simulink model "Sinusoidal_Road"  (R2023b)
settings: Solver=VariableStepAuto  StartTime=0.0  StopTime=10  RelTol=1e-3
values from neighbouring files (symbols this model uses):
  A = [0.01, 0.05, 0.1]    [Parameters.m]
  a = 1.35    [Parameters.m]
  b = 1.5    [Parameters.m]
  g = 9.81    [Parameters.m]
  I = 650    [Parameters.m]
  Kt = 14e4    (= 140000)    [Parameters.m]
  lambda = 1    [Parameters.m]
  Mw = 20    [Parameters.m]
  v = [1, 2, 3, 5, 8, 10]    [Parameters.m]
libraries: CarModelLibrary x6, simulink x4
settings Model: Creator=fb552  LastModifiedBy=franc
settings SolverCC: AlgebraicLoopSolver=TrustRegion
settings DebuggingCC: UnconnectedInputMsg=warning  UnconnectedOutputMsg=warning  UnconnectedLineMsg=warning
settings ModelReferenceCC: EnableRefExpFcnMdlSchedulingChecks=on

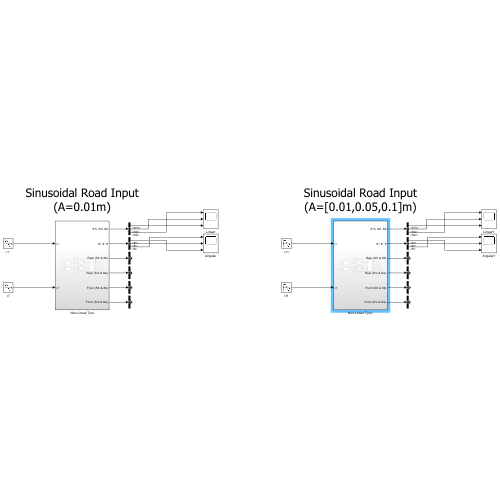
[thumbnail: Simulink's stored preview of the top-level diagram]
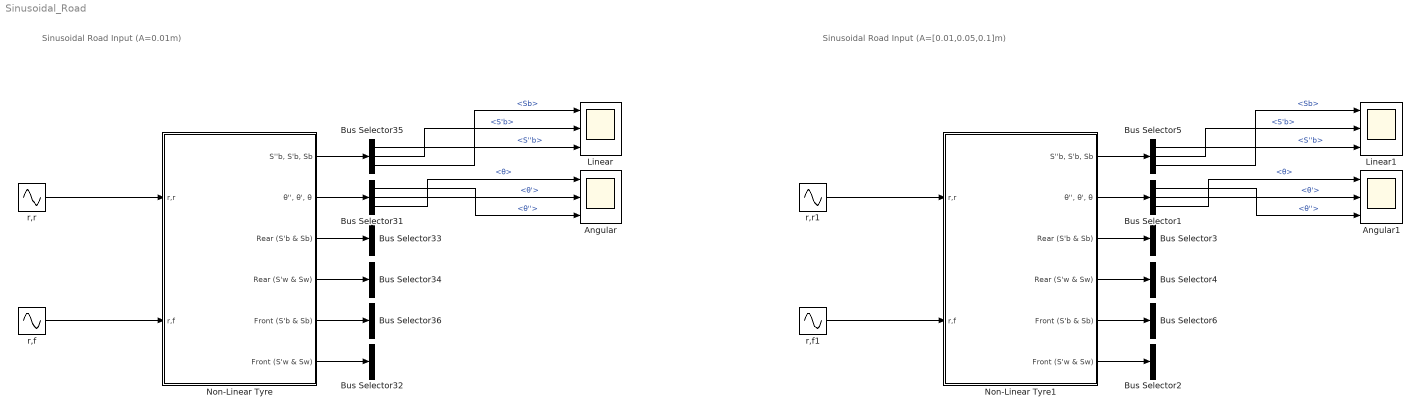
== system Sinusoidal_Road ==
  note: Sinusoidal Road Input (A=0.01m)
  note: Sinusoidal Road Input (A=[0.01,0.05,0.1]m)
  Angular : Scope  NumInputPorts=3
  Angular1 : Scope  NumInputPorts=3
  Bus Selector1 : BusSelector  OutputSignals=θ'',θ',θ
  Bus Selector{2,4,32,34} (4 alike) : BusSelector  OutputSignals=Sw
  Bus Selector{3,6,33,36} (4 alike) : BusSelector  OutputSignals=Sb
  Bus Selector31 : BusSelector  OutputSignals=θ'',θ',θ
  Bus Selector35 : BusSelector  OutputSignals=S''b,S'b,Sb
  Bus Selector5 : BusSelector  OutputSignals=S''b,S'b,Sb
  Linear : Scope  NumInputPorts=3
  Linear1 : Scope  NumInputPorts=3
  Non-Linear Tyre : Subsystem
  Non-Linear Tyre1 : Subsystem
  r,f : Sin  Amplitude=A(1)  Frequency=2*pi*(v/lambda)  SampleTime=0
  r,f1 : Sin  Amplitude=A  Frequency=2*pi*(v(end)/lambda)  SampleTime=0
  r,r : Sin  Amplitude=A(1)  Frequency=2*pi*(v/lambda)  Phase=(a+b)*2*pi  SampleTime=0
  r,r1 : Sin  Amplitude=A  Frequency=2*pi*(v(end)/lambda)  Phase=(a+b)*2*pi  SampleTime=0
  wires:
  Non-Linear Tyre/2("θ'', θ', θ") -> Bus Selector31/1
  Non-Linear Tyre/6(Front (S'w & Sw)) -> Bus Selector32/1
  Bus Selector35/3 -> Linear/1  "<Sb>"
  Non-Linear Tyre/4(Rear (S'w & Sw)) -> Bus Selector34/1
  Non-Linear Tyre/5(Front (S'b & Sb)) -> Bus Selector36/1
  Non-Linear Tyre/1("S''b, S'b, Sb") -> Bus Selector35/1
  Non-Linear Tyre/3(Rear (S'b & Sb)) -> Bus Selector33/1
  r,f/1 -> Non-Linear Tyre/2(r,f)
  r,r/1 -> Non-Linear Tyre/1(r,r)
  Bus Selector35/2 -> Linear/2  "<S'b>"
  Bus Selector35/1 -> Linear/3  "<S''b>"
  Bus Selector31/3 -> Angular/1  "<θ>"
  Bus Selector31/2 -> Angular/2  "<θ'>"
  Bus Selector31/1 -> Angular/3  "<θ''>"
  Non-Linear Tyre1/3(Rear (S'b & Sb)) -> Bus Selector3/1
  Bus Selector5/3 -> Linear1/1  "<Sb>"
  r,r1/1 -> Non-Linear Tyre1/1(r,r)
  Bus Selector5/2 -> Linear1/2  "<S'b>"
  r,f1/1 -> Non-Linear Tyre1/2(r,f)
  Non-Linear Tyre1/2("θ'', θ', θ") -> Bus Selector1/1
  Non-Linear Tyre1/4(Rear (S'w & Sw)) -> Bus Selector4/1
  Non-Linear Tyre1/5(Front (S'b & Sb)) -> Bus Selector6/1
  Bus Selector1/3 -> Angular1/1  "<θ>"
  Non-Linear Tyre1/1("S''b, S'b, Sb") -> Bus Selector5/1
  Bus Selector1/1 -> Angular1/3  "<θ''>"
  Bus Selector1/2 -> Angular1/2  "<θ'>"
  Non-Linear Tyre1/6(Front (S'w & Sw)) -> Bus Selector2/1
  Bus Selector5/1 -> Linear1/3  "<S''b>"

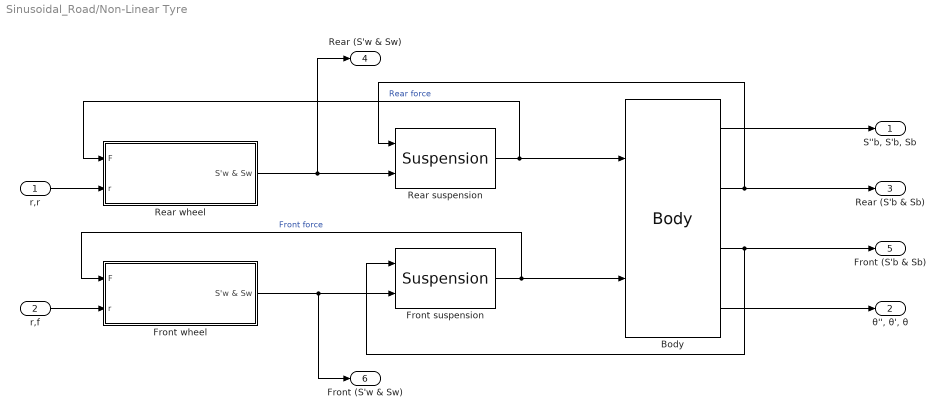
== system Sinusoidal_Road/Non-Linear Tyre ==
  r,r : Inport
  r,f : Inport  Port=2
  Body : CarModelLibrary/Body  mb=Mb  I=I  a=a  b=b
  Front suspension : CarModelLibrary/Suspension  ks=Ks  ksstiff=Kstiff  x0=x0  csb=Csc  csr=Cse
  Front wheel : Subsystem  AncestorBlock=CarModelLibrary/Wheel  mask{mw=Mw, Kt=Kt, g=g}
      mask prompts: mw "Wheel Mass (Kg)"; Kt "Tyre Stiffness"; g "Gravitational acceleration"
  Rear suspension : CarModelLibrary/Suspension  ks=Ks  ksstiff=Kstiff  x0=x0  csb=Csc  csr=Cse
  Rear wheel : Subsystem  AncestorBlock=CarModelLibrary/Wheel  mask{mw=Mw, Kt=Kt, g=g}
      mask prompts: mw "Wheel Mass (Kg)"; Kt "Tyre Stiffness"; g "Gravitational acceleration"
  "S''b, S'b, Sb" : Outport
  "θ'', θ', θ" : Outport  Port=2
  Rear (S'b & Sb) : Outport  Port=3
  Rear (S'w & Sw) : Outport  Port=4
  Front (S'b & Sb) : Outport  Port=5
  Front (S'w & Sw) : Outport  Port=6
  wires:
  Body/1 -> "S''b, S'b, Sb"/1
  Body/2 -> Rear suspension/1, Rear (S'b & Sb)/1
  Front wheel/1(S'w & Sw) -> Front suspension/2, Front (S'w & Sw)/1
  Rear wheel/1(S'w & Sw) -> Rear suspension/2, Rear (S'w & Sw)/1
  Body/4 -> "θ'', θ', θ"/1
  Body/3 -> Front suspension/1, Front (S'b & Sb)/1
  Rear suspension/1 -> Body/1, Rear wheel/1(F)  "Rear force"
  r,r/1 -> Rear wheel/2(r)
  r,f/1 -> Front wheel/2(r)
  Front suspension/1 -> Front wheel/1(F), Body/2  "Front force"

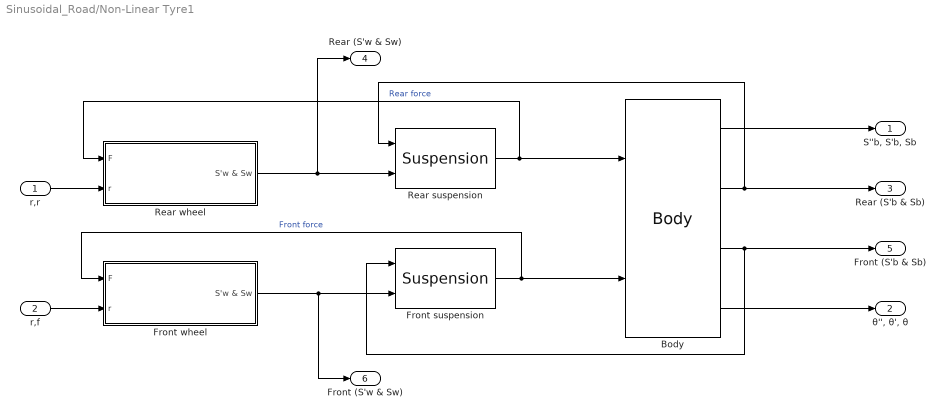
== system Sinusoidal_Road/Non-Linear Tyre1 ==
  r,r : Inport
  r,f : Inport  Port=2
  Body : CarModelLibrary/Body  mb=Mb  I=I  a=a  b=b
  Front suspension : CarModelLibrary/Suspension  ks=Ks  ksstiff=Kstiff  x0=x0  csb=Csc  csr=Cse
  Front wheel : Subsystem  AncestorBlock=CarModelLibrary/Wheel  mask{mw=Mw, Kt=Kt, g=g}
      mask prompts: mw "Wheel Mass (Kg)"; Kt "Tyre Stiffness"; g "Gravitational acceleration"
  Rear suspension : CarModelLibrary/Suspension  ks=Ks  ksstiff=Kstiff  x0=x0  csb=Csc  csr=Cse
  Rear wheel : Subsystem  AncestorBlock=CarModelLibrary/Wheel  mask{mw=Mw, Kt=Kt, g=g}
      mask prompts: mw "Wheel Mass (Kg)"; Kt "Tyre Stiffness"; g "Gravitational acceleration"
  "S''b, S'b, Sb" : Outport
  "θ'', θ', θ" : Outport  Port=2
  Rear (S'b & Sb) : Outport  Port=3
  Rear (S'w & Sw) : Outport  Port=4
  Front (S'b & Sb) : Outport  Port=5
  Front (S'w & Sw) : Outport  Port=6
  wires:
  Body/1 -> "S''b, S'b, Sb"/1
  Body/2 -> Rear suspension/1, Rear (S'b & Sb)/1
  Front wheel/1(S'w & Sw) -> Front suspension/2, Front (S'w & Sw)/1
  Rear wheel/1(S'w & Sw) -> Rear suspension/2, Rear (S'w & Sw)/1
  Body/4 -> "θ'', θ', θ"/1
  Body/3 -> Front suspension/1, Front (S'b & Sb)/1
  Rear suspension/1 -> Body/1, Rear wheel/1(F)  "Rear force"
  r,r/1 -> Rear wheel/2(r)
  r,f/1 -> Front wheel/2(r)
  Front suspension/1 -> Front wheel/1(F), Body/2  "Front force"

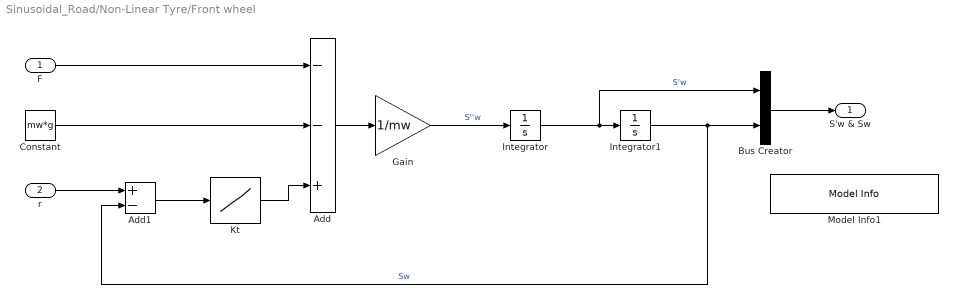
== system Sinusoidal_Road/Non-Linear Tyre/Front wheel ==
  F : Inport
  r : Inport  Port=2
  Add : Sum  Inputs=--+
  Add1 : Sum  Inputs=+-
  Bus Creator : BusCreator  Inputs=2
  Constant : Constant  Value=mw*g
  Gain : Gain  Gain=1/mw
  Integrator : Integrator
  Integrator1 : Integrator
  Kt : Lookup_n-D  NumberOfTableDimensions=1  BreakpointsForDimension1=[-1, 0, 1]  Table=[0, 0, Kt]  InternalRulePriority=Speed  RndMeth=Simplest
  Model Info1 : simulink/Model-Wide Utilities/Model Info  Frame=on  DisplayStringWithTags=m * S''w = -F + Kt (r-S) - m*g  HorizontalTextAlignment=Center  LeftAlignmentValue=0.5
  S'w & Sw : Outport
  wires:
  Kt/1 -> Add/3
  F/1 -> Add/1
  Constant/1 -> Add/2
  Gain/1 -> Integrator/1  "S''w"
  Add/1 -> Gain/1
  Integrator1/1 -> Add1/2, Bus Creator/2  "Sw"
  Bus Creator/1 -> S'w & Sw/1
  Integrator/1 -> Integrator1/1, Bus Creator/1  "S'w"
  Add1/1 -> Kt/1
  r/1 -> Add1/1

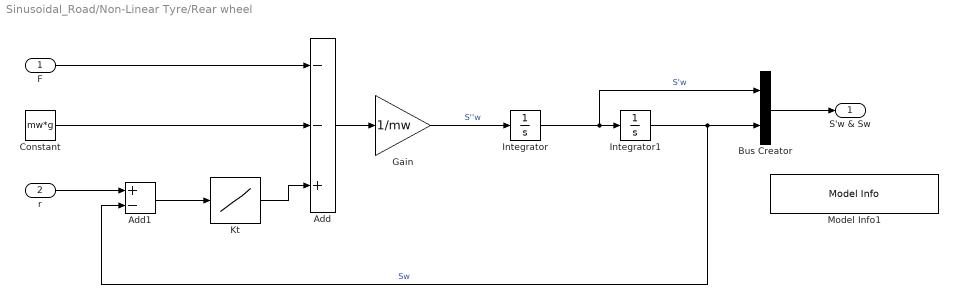
== system Sinusoidal_Road/Non-Linear Tyre/Rear wheel ==
  F : Inport
  r : Inport  Port=2
  Add : Sum  Inputs=--+
  Add1 : Sum  Inputs=+-
  Bus Creator : BusCreator  Inputs=2
  Constant : Constant  Value=mw*g
  Gain : Gain  Gain=1/mw
  Integrator : Integrator
  Integrator1 : Integrator
  Kt : Lookup_n-D  NumberOfTableDimensions=1  BreakpointsForDimension1=[-1, 0, 1]  Table=[0, 0, Kt]  InternalRulePriority=Speed  RndMeth=Simplest
  Model Info1 : simulink/Model-Wide Utilities/Model Info  Frame=on  DisplayStringWithTags=m * S''w = -F + Kt (r-S) - m*g  HorizontalTextAlignment=Center  LeftAlignmentValue=0.5
  S'w & Sw : Outport
  wires:
  Kt/1 -> Add/3
  F/1 -> Add/1
  Constant/1 -> Add/2
  Gain/1 -> Integrator/1  "S''w"
  Add/1 -> Gain/1
  Integrator1/1 -> Add1/2, Bus Creator/2  "Sw"
  Bus Creator/1 -> S'w & Sw/1
  Integrator/1 -> Integrator1/1, Bus Creator/1  "S'w"
  Add1/1 -> Kt/1
  r/1 -> Add1/1

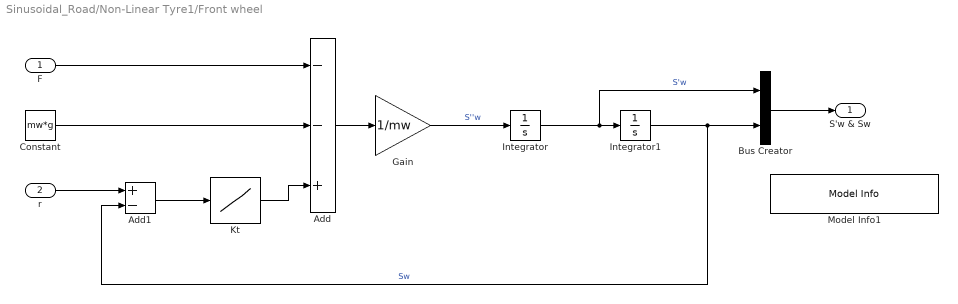
== system Sinusoidal_Road/Non-Linear Tyre1/Front wheel ==
  F : Inport
  r : Inport  Port=2
  Add : Sum  Inputs=--+
  Add1 : Sum  Inputs=+-
  Bus Creator : BusCreator  Inputs=2
  Constant : Constant  Value=mw*g
  Gain : Gain  Gain=1/mw
  Integrator : Integrator
  Integrator1 : Integrator
  Kt : Lookup_n-D  NumberOfTableDimensions=1  BreakpointsForDimension1=[-1, 0, 1]  Table=[0, 0, Kt]  InternalRulePriority=Speed  RndMeth=Simplest
  Model Info1 : simulink/Model-Wide Utilities/Model Info  Frame=on  DisplayStringWithTags=m * S''w = -F + Kt (r-S) - m*g  HorizontalTextAlignment=Center  LeftAlignmentValue=0.5
  S'w & Sw : Outport
  wires:
  Kt/1 -> Add/3
  F/1 -> Add/1
  Constant/1 -> Add/2
  Gain/1 -> Integrator/1  "S''w"
  Add/1 -> Gain/1
  Integrator1/1 -> Add1/2, Bus Creator/2  "Sw"
  Bus Creator/1 -> S'w & Sw/1
  Integrator/1 -> Integrator1/1, Bus Creator/1  "S'w"
  Add1/1 -> Kt/1
  r/1 -> Add1/1

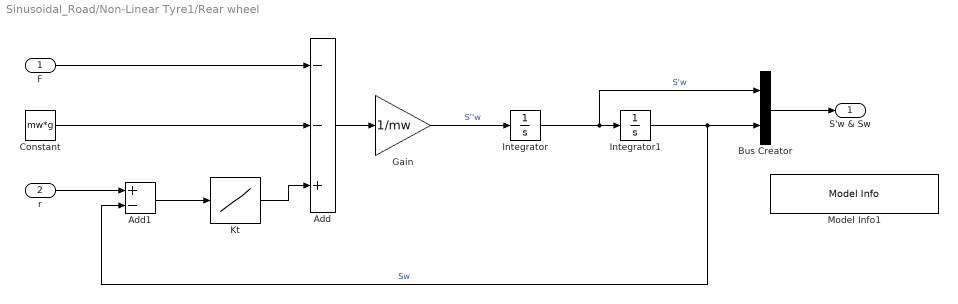
== system Sinusoidal_Road/Non-Linear Tyre1/Rear wheel ==
  F : Inport
  r : Inport  Port=2
  Add : Sum  Inputs=--+
  Add1 : Sum  Inputs=+-
  Bus Creator : BusCreator  Inputs=2
  Constant : Constant  Value=mw*g
  Gain : Gain  Gain=1/mw
  Integrator : Integrator
  Integrator1 : Integrator
  Kt : Lookup_n-D  NumberOfTableDimensions=1  BreakpointsForDimension1=[-1, 0, 1]  Table=[0, 0, Kt]  InternalRulePriority=Speed  RndMeth=Simplest
  Model Info1 : simulink/Model-Wide Utilities/Model Info  Frame=on  DisplayStringWithTags=m * S''w = -F + Kt (r-S) - m*g  HorizontalTextAlignment=Center  LeftAlignmentValue=0.5
  S'w & Sw : Outport
  wires:
  Kt/1 -> Add/3
  F/1 -> Add/1
  Constant/1 -> Add/2
  Gain/1 -> Integrator/1  "S''w"
  Add/1 -> Gain/1
  Integrator1/1 -> Add1/2, Bus Creator/2  "Sw"
  Bus Creator/1 -> S'w & Sw/1
  Integrator/1 -> Integrator1/1, Bus Creator/1  "S'w"
  Add1/1 -> Kt/1
  r/1 -> Add1/1
